simulink model "qam_64_constellation"  (R2019b)
settings: Solver=VariableStepAuto  StartTime=0.0  StopTime=10.0  RelTol=1e-3
libraries: commdigbbndam3 x2, commchan3 x1, commsink2 x1, commrandsrc2 x1
settings Model: Creator=janic  LastModifiedBy=janic

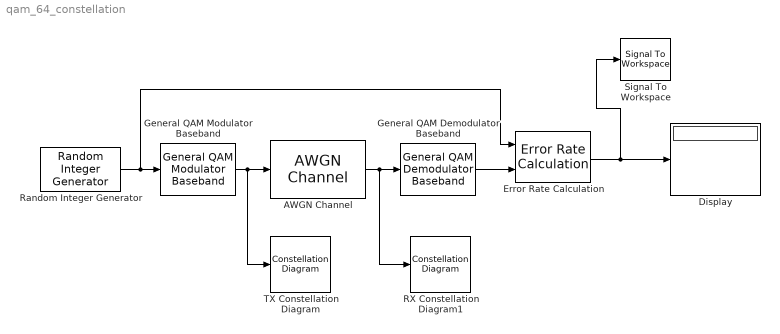
== system qam_64_constellation ==
  AWGN Channel : commchan3/AWGN Channel  InputProcessing=Columns as channels (frame based)  seed=67  noiseMode="Signal to noise ratio  (Eb/No)"  EbNodB=6  EsNodB=10  SNRdB=10  bitsPerSym=2  Ps=1  Tsym=1  variance=1
      settings: SourceProductName=Communications Toolbox
  Display : Display
  Error Rate Calculation : commsink2/Error Rate Calculation  N=0  st_delay=0  cp_mode=Entire frame  subframe=[]  PMode=Port  WsName=ErrorVec  RsMode2=off  stop=on  numErr=1000  maxBits=1e8
      settings: SourceProductName=Communications Toolbox
  General QAM Demodulator Baseband : commdigbbndam3/General QAM Demodulator Baseband  SigCon=[exp(2*pi*1i*[0:63]/64)]  OutType=Integer  DecType=Hard decision  VarSource=Dialog  Variance=1  outDtypeBit=Inherit via internal rule  outDtype=Inherit via internal rule  roundingMode=Floor  overflowMode=Wrap  OvFlMode=off  OvFlModeLastStrValue=off  sigConstWordLen=16  sigConstDataTypeStr=Inherit: Same word length as input  sigConstLastDataTypeStr=Inherit: Same word length as input  accum1WordLen=32  accum1FracLen=30  prodInWordLen=32  prodInFracLen=30  prodInDataTypeStr=Inherit: Same as accumulator 1  prodInLastDataTypeStr=Inherit: Same as accumulator 1  prodOutWordLen=32  prodOutFracLen=30  accum2WordLen=32  accum2FracLen=30  accum3WordLen=32  accum3FracLen=30  nsiWordLen=32  nsiFracLen=30  nsiDataTypeStr=Inherit: Same as accumulator 3  nsiLastDataTypeStr=Inherit: Same as accumulator 3  invn0WordLen=16  invn0FracLen=8  invn0DataTypeStr=Inherit: Same word length as input  invn0LastDataTypeStr=Inherit: Same word length as input  outputWordLen=32  outputFracLen=30
      settings: SourceProductName=Communications Toolbox  SourceProductBaseCode=CM
  General QAM Modulator Baseband : commdigbbndam3/General QAM Modulator Baseband  SigCon=[exp(2*pi*1i*[0:63]/64)]  outDtype=double  outWordLen=16  outUDDataType=sfix(16)  outFracLenMode=Best precision  outFracLen=15  outDataTypeStr=double  outLastDataTypeStr=double
      settings: SourceProductName=Communications Toolbox  SourceProductBaseCode=CM
  RX Constellation Diagram1 : ConstellationDiagram
  Random Integer Generator : commrandsrc2/Random Integer Generator  mul=4  seed=37  Ts=1  frameBased=on  sampPerFrame=1000  orient=off  outDataType=double
      settings: SourceProductName=Communications Toolbox  SourceProductBaseCode=CM
  Signal To Workspace : SignalToWorkspace  VariableName=BER
      settings: CopyFcn=dspblkcopystw(gcbh);  MaxDataPoints=1
  TX Constellation Diagram : ConstellationDiagram
  wires:
  General QAM Modulator Baseband/1 -> AWGN Channel/1, TX Constellation Diagram/1
  General QAM Demodulator Baseband/1 -> Error Rate Calculation/2
  AWGN Channel/1 -> General QAM Demodulator Baseband/1, RX Constellation Diagram1/1
  Random Integer Generator/1 -> General QAM Modulator Baseband/1, Error Rate Calculation/1
  Error Rate Calculation/1 -> Signal To Workspace/1, Display/1
